simulink model "main_sim_adapt"  (Simulink 7.2)
settings: Solver=ode2  SolverMode=SingleTasking  StartTime=0.0  StopTime=tsim_max  FixedStep=dtsim  RelTol=1e-3
StopFcn:
  | %mkplt
undefined symbols (not defined in the file): aero_surf_qbar_off, aero_surf_qbar_on, assertion_time, att_type, att_type_numbers, bb_ellipsoid, bb_params, compute_all_rate_cols, compute_all_vel_cols, constants, cosA, DiscIntNeverNeededParam, dtsim, E_rwy, eow_boundary, full_surf_llim, full_surf_ulim, gain_set, gain_var_struct, in_exsig_vecin, in_exsig_vecout, MACH, MACH_att_fb, MACH_gain_mat, MACH_mass_IC, MACH_pos_IC, MACH_pqr_Bmat_IC, MACH_pqr_IC, MACH_pqr_u_IC, MACH_quat_IC, MACH_throttle_IC, MACH_U_nom_IC, MACH_vel_Bmat_IC, MACH_vel_cvdnom_IC, MACH_vel_IC, MACH_vel_uold_IC, max_LOS_rate, modes, N_rwy, pos, rcs_cvddes_thresh, reset_camcmd_on_entry, sinA, target_pos_IC, target_range_blind, target_range_detect, target_range_homing, target_vel_IC, trac_params, u_llim, u_ulim, use_auto_att_type, use_eow_as_iv, use_nav, use_pos_fltpath_lim, use_throt_estimate, use_variable_mass, use_wind_est, vel, vel_cmd_ramp_time ... (+1)
libraries: simulink x32, mach_lib x26, utility_lib x24, model_lib x15, simulink_need_slupdate x8, models x6
(part 5 of 5)

== system main_sim_adapt/claw_main/vel_loops/set di params/compute dc_fltpath ==
  NEh_dot_fltpath : Inport  OutDataType=sfix(16)  OutScaling=2^0
  Gain : Gain  Gain=repmat([1 1 -1],3,1)  ParameterDataType=sfix(16)  ParameterScaling=2^0  OutDataType=sfix(16)  OutScaling=2^0
  Gain1 : Gain  Gain=[1 1 -1]  ParameterDataType=sfix(16)  ParameterScaling=2^0  OutDataType=sfix(16)  OutScaling=2^0
  Reshape : Reshape  OutputDimensionality=Customize  OutputDimensions=[3 3]
  Terminator : Terminator
  vec2dc : utility_lib/vec2dc  SystemSampleTime=-1
  dc_fltpath : Outport  OutDataType=sfix(16)  OutScaling=2^0
  wires:
  vec2dc/1 -> Reshape/1
  Reshape/1 -> Gain/1
  Gain1/1 -> vec2dc/1
  vec2dc/2 -> Terminator/1
  Gain/1 -> dc_fltpath/1
  NEh_dot_fltpath/1 -> Gain1/1

== system main_sim_adapt/claw_main/vel_loops/set di params/throttle limits ==
  full_surf : Inport  OutDataType=sfix(16)  OutScaling=2^0
  throt_old : Inport  Port=2  OutDataType=sfix(16)  OutScaling=2^0
  Bus Creator : BusCreator
  Bus Selector1 : BusSelector  OutputSignals=full_surf_ulim,full_surf_llim,full_surf_urlim,full_surf_lrlim
  Selector{1..2,5..6} (4 alike) : Selector  InputPortWidth=MACH.num_u  IndexOptions=Index vector (dialog)  Indices=MACH.throttle_idx  OutputSizes=1
  rate limit limits : mach_lib/rate limit limits  SystemSampleTime=-1  ulim=MACH.vel_throt_ulim  llim=MACH.vel_throt_llim
  throt_limits : Outport  OutDataType=sfix(16)  OutScaling=2^0
  wires:
  Bus Selector1/1 -> Selector5/1  "<full_surf_ulim>"
  Bus Selector1/2 -> Selector6/1  "<full_surf_llim>"
  full_surf/1 -> Bus Selector1/1
  throt_old/1 -> rate limit limits/1
  Selector5/1 -> rate limit limits/2
  Selector6/1 -> rate limit limits/3
  Bus Creator/1 -> throt_limits/1
  rate limit limits/1 -> Bus Creator/1  "throt_ulim"
  rate limit limits/2 -> Bus Creator/2  "throt_llim"
  Bus Selector1/3 -> Selector1/1  "<full_surf_urlim>"
  Bus Selector1/4 -> Selector2/1  "<full_surf_lrlim>"
  Selector1/1 -> rate limit limits/4, Bus Creator/3  "throt_urlim"
  Selector2/1 -> rate limit limits/5, Bus Creator/4  "throt_lrlim"

== system main_sim_adapt/vehicle_model/target/seeker model/seeker model/cart to polar ==
  note: Avoid division by zero when
      | all errors are exactly zero
  scaling info : Inport  OutDataType=sfix(16)  OutScaling=2^0
  cross_d;vert_d : Inport  Port=2  OutDataType=sfix(16)  OutScaling=2^0
  Abs : Abs
  Bus Selector : BusSelector  OutputSignals=Rground,Rslant
  Constant : Constant  Value=0.0001  OutDataType=sfix(16)  OutScaling=2^0
  Gain1 : Gain  Gain=1./max_LOS_rate  ParameterDataType=sfix(16)  ParameterScaling=2^0  OutDataType=sfix(16)  OutScaling=2^0
  Gain2 : Gain  Gain=[1 -1]  ParameterDataType=sfix(16)  ParameterScaling=2^0  OutDataType=sfix(16)  OutScaling=2^0
  MinMax : MinMax  Function=max  Inputs=3  OutDataType=sfix(16)  OutScaling=2^0
  Mux : Mux  Inputs=2
  Product : Product  Inputs=*/  OutDataType=sfix(16)  OutScaling=2^0  RndMeth=Zero
  LOS_rate : Outport  OutDataType=sfix(16)  OutScaling=2^0
  wires:
  Mux/1 -> MinMax/2
  Gain1/1 -> MinMax/1
  Gain2/1 -> Product/2
  MinMax/1 -> Gain2/1
  Abs/1 -> Gain1/1
  Product/1 -> LOS_rate/1
  cross_d;vert_d/1 -> Product/1, Abs/1
  scaling info/1 -> Bus Selector/1
  Bus Selector/1 -> Mux/1  "<Rground>"
  Bus Selector/2 -> Mux/2  "<Rslant>"
  Constant/1 -> MinMax/3

== system main_sim_adapt/claw_main/input processing/mode dependent stick processing/att rate cmd/also reset att on att_type change ==
  reset_in : Inport  OutDataType=sfix(16)  OutScaling=2^0
  Detect Change : simulink/Logic and Bit Operations/Detect Change  SystemSampleTime=-1  vinit=0
  Detect Increase : simulink/Logic and Bit Operations/Detect Increase  SystemSampleTime=-1  vinit=0.0
  Logical Operator2 : Logic  Operator=OR  AllPortsSameDT=off
  Logical Operator3 : Logic  Operator=XOR  AllPortsSameDT=off
  Unit Delay : UnitDelay  Orientation=left  SampleTime=MACH.dt
  reset_out : Outport  OutDataType=sfix(16)  OutScaling=2^0
  wires:
  [att_type] -> Detect Change/1
  Detect Change/1 -> Logical Operator2/2
  Detect Increase/1 -> Logical Operator2/1
  Logical Operator2/1 -> Logical Operator3/1
  Logical Operator3/1 -> Unit Delay/1, reset_out/1
  Unit Delay/1 -> Logical Operator3/2
  reset_in/1 -> Detect Increase/1

== system main_sim_adapt/claw_main/input processing/mode dependent stick processing/feed forward/get att_ff ==
  signal_bus : Inport  OutDataType=sfix(16)  OutScaling=2^0
  Bus Selector : BusSelector  OutputSignals=x_est.uvw,y_meas.accels_cg,y_meas.dircos,x_est.e
  Dot Product : simulink/Math Operations/Dot Product  InputSameDT=on  OutDataType=sfix(16)  OutScaling=2^-10  DoSatur=off
  Gain : Gain  Gain=constants.g  ParameterDataType=sfix(16)  ParameterScaling=2^0  OutDataType=sfix(16)  OutScaling=2^0
  MinMax1 : MinMax  Function=max  Inputs=2  OutDataType=sfix(16)  OutScaling=2^0
  Product1 : Product  Inputs=/*  OutDataType=sfix(16)  OutScaling=2^0  RndMeth=Zero
  Sum2 : Sum  Inputs=|++  OutDataType=sfix(16)  OutScaling=2^0
  V x a : utility_lib/cross product  SystemSampleTime=-1
  down vector : Selector  InputPortWidth=9  IndexOptions=Index vector (dialog)  Indices=7:9  OutputSizes=1
  geted : utility_lib/geted  SystemSampleTime=-1
  protect for   divide by zero : Constant  Value=0.001^2  OutDataType=sfix(16)  OutScaling=2^0
  att_ff : Outport  OutDataType=sfix(16)  OutScaling=2^0
  wires:
  Product1/1 -> geted/1
  V x a/1 -> Product1/2
  signal_bus/1 -> Bus Selector/1
  Bus Selector/1 -> V x a/1, Dot Product/1, Dot Product/2  "<uvw>"
  Bus Selector/4 -> geted/2  "<e>"
  protect for   divide by zero/1 -> MinMax1/2
  MinMax1/1 -> Product1/1
  Sum2/1 -> V x a/2
  geted/1 -> att_ff/1
  Bus Selector/3 -> down vector/1  "<dircos>"
  down vector/1 -> Gain/1
  Gain/1 -> Sum2/2
  Bus Selector/2 -> Sum2/1  "<accels_cg>"
  Dot Product/1 -> MinMax1/1

== system main_sim_adapt/claw_main/input processing/mode dependent stick processing/feed forward/lookup using  energy over weight ==
  eow_idx : Inport  OutDataType=sfix(16)  OutScaling=2^0
  Constant1 : Constant  Value=int32(0:2)  OutDataType=sfix(16)  OutScaling=2^0
  Constant2 : Constant  Value=int32(0:2)  OutDataType=sfix(16)  OutScaling=2^0
  Interpolation (n-D) using PreLookup for acc : simulink_need_slupdate/Interpolation (n-D) using PreLookup  numDimsPopupSelect=2  explicitNumDims=2  table=tbl_acc_eow  interpMethod=Linear  extrapMethod=Linear  rangeErrorMode=None  NumSelectionDims=1
  Interpolation (n-D) using PreLookup for vel : simulink_need_slupdate/Interpolation (n-D) using PreLookup  numDimsPopupSelect=2  explicitNumDims=2  table=tbl_vel_eow  interpMethod=Linear  extrapMethod=Linear  rangeErrorMode=None  NumSelectionDims=1
  pos_ff : Outport  OutDataType=sfix(16)  OutScaling=2^0
  vel_ff : Outport  Port=2  OutDataType=sfix(16)  OutScaling=2^0
  wires:
  Interpolation (n-D) using PreLookup for vel/1 -> pos_ff/1
  Interpolation (n-D) using PreLookup for acc/1 -> vel_ff/1
  eow_idx/1 -> Interpolation (n-D) using PreLookup for vel/1, Interpolation (n-D) using PreLookup for acc/1
  Constant1/1 -> Interpolation (n-D) using PreLookup for vel/2
  Constant2/1 -> Interpolation (n-D) using PreLookup for acc/2

== system main_sim_adapt/claw_main/input processing/mode dependent stick processing/feed forward/lookup using X   ==
  X_idx : Inport  OutDataType=sfix(16)  OutScaling=2^0
  Constant1 : Constant  Value=int32(0:2)  OutDataType=sfix(16)  OutScaling=2^0
  Constant2 : Constant  Value=int32(0:2)  OutDataType=sfix(16)  OutScaling=2^0
  Interpolation (n-D) using PreLookup for acc : simulink_need_slupdate/Interpolation (n-D) using PreLookup  numDimsPopupSelect=2  explicitNumDims=2  table=tbl_acc_X  interpMethod=Linear  extrapMethod=Linear  rangeErrorMode=None  NumSelectionDims=1
  Interpolation (n-D) using PreLookup for vel : simulink_need_slupdate/Interpolation (n-D) using PreLookup  numDimsPopupSelect=2  explicitNumDims=2  table=tbl_vel_X  interpMethod=Linear  extrapMethod=Linear  rangeErrorMode=None  NumSelectionDims=1
  pos_ff : Outport  OutDataType=sfix(16)  OutScaling=2^0
  vel_ff : Outport  Port=2  OutDataType=sfix(16)  OutScaling=2^0
  wires:
  X_idx/1 -> Interpolation (n-D) using PreLookup for vel/1, Interpolation (n-D) using PreLookup for acc/1
  Interpolation (n-D) using PreLookup for vel/1 -> pos_ff/1
  Interpolation (n-D) using PreLookup for acc/1 -> vel_ff/1
  Constant1/1 -> Interpolation (n-D) using PreLookup for vel/2
  Constant2/1 -> Interpolation (n-D) using PreLookup for acc/2

== system main_sim_adapt/claw_main/input processing/mode dependent stick processing/set command selection switches/modify for accel cmd submode ==
  select_cmd_in : Inport  OutDataType=sfix(16)  OutScaling=2^0
  accel_cmd_sw : Inport  Port=2  OutDataType=sfix(16)  OutScaling=2^0
  Assignment : Assignment  IndexOptions=Index vector (dialog)  Indices=[1 2 4]  OutputSizes=[1 1]
  Assignment1 : Assignment  IndexOptions=Index vector (dialog)  Indices=[1 2 4]  OutputSizes=[1 1]
  Bus Assignment : BusAssignment  AssignedSignals=vel,pos
  Bus Selector : BusSelector  OutputSignals=vel
  Bus Selector1 : BusSelector  OutputSignals=pos
  Selector1 : Selector  InputPortWidth=4  IndexOptions=Index vector (dialog)  Indices=[1 2 4]  OutputSizes=1
  Selector2 : Selector  InputPortWidth=4  IndexOptions=Index vector (dialog)  Indices=[1 2 4]  OutputSizes=1
  Switch : Switch  Threshold=0.5
  Switch1 : Switch  Threshold=0.5
  command current pos : Constant  Value=0  OutDataType=sfix(16)  OutScaling=2^0
  command current vel : Constant  Value=0  OutDataType=sfix(16)  OutScaling=2^0
  select_cmd : Outport  OutDataType=sfix(16)  OutScaling=2^0
  wires:
  select_cmd_in/1 -> Bus Assignment/1, Bus Selector/1, Bus Selector1/1
  accel_cmd_sw/1 -> Switch/2, Switch1/2
  Bus Selector/1 -> Selector1/1, Assignment/1  "<vel>"
  command current vel/1 -> Switch/1
  Selector1/1 -> Switch/3
  Switch/1 -> Assignment/2
  Assignment/1 -> Bus Assignment/2
  Bus Assignment/1 -> select_cmd/1
  Bus Selector1/1 -> Selector2/1, Assignment1/1  "<pos>"
  command current pos/1 -> Switch1/1
  Selector2/1 -> Switch1/3
  Switch1/1 -> Assignment1/2
  Assignment1/1 -> Bus Assignment/3

== system main_sim_adapt/claw_main/input processing/mode dependent stick processing/use table lookup pos cmds/use E/W to get pos cmds ==
  eow_idx : Inport  OutDataType=sfix(16)  OutScaling=2^0
  Constant1 : Constant  Value=int32(0:2)  OutDataType=sfix(16)  OutScaling=2^0
  Interpolation (n-D) using PreLookup : simulink_need_slupdate/Interpolation (n-D) using PreLookup  numDimsPopupSelect=2  explicitNumDims=2  table=tbl_pos_eow  interpMethod=Linear  extrapMethod=Linear  rangeErrorMode=None  NumSelectionDims=1
  pos_cmd_eow : Outport  OutDataType=sfix(16)  OutScaling=2^0
  wires:
  Interpolation (n-D) using PreLookup/1 -> pos_cmd_eow/1
  eow_idx/1 -> Interpolation (n-D) using PreLookup/1
  Constant1/1 -> Interpolation (n-D) using PreLookup/2

== system main_sim_adapt/claw_main/input processing/mode dependent stick processing/use table lookup pos cmds/use X to get pos cmds ==
  note: Note: When X is used as the independent variable
      | the trajectory is in a vertical plane and Y=0
  X_idx : Inport  OutDataType=sfix(16)  OutScaling=2^0
  X : Inport  Port=2  OutDataType=sfix(16)  OutScaling=2^0
  Constant1 : Constant  Value=E_rwy  OutDataType=sfix(16)  OutScaling=2^0
  Constant3 : Constant  Value=N_rwy  OutDataType=sfix(16)  OutScaling=2^0
  Constant4 : Constant  Value=cosA  OutDataType=sfix(16)  OutScaling=2^0
  Constant5 : Constant  Value=sinA  OutDataType=sfix(16)  OutScaling=2^0
  Interpolation (n-D) using PreLookup for h : simulink_need_slupdate/Interpolation (n-D) using PreLookup  numDimsPopupSelect=1  explicitNumDims=2  table=tbl_hofX  interpMethod=Linear  extrapMethod=Linear  rangeErrorMode=None  NumSelectionDims=0
  Mux : Mux  Inputs=3
  Product3 : Product  OutDataType=sfix(16)  OutScaling=2^0  RndMeth=Zero
  Product4 : Product  OutDataType=sfix(16)  OutScaling=2^0  RndMeth=Zero
  Sum4 : Sum  Inputs=++|  OutDataType=sfix(16)  OutScaling=2^0
  Sum5 : Sum  Inputs=|++  OutDataType=sfix(16)  OutScaling=2^0
  pos_cmd_X : Outport  OutDataType=sfix(16)  OutScaling=2^0
  wires:
  X_idx/1 -> Interpolation (n-D) using PreLookup for h/1
  Interpolation (n-D) using PreLookup for h/1 -> Mux/3
  Mux/1 -> pos_cmd_X/1
  Constant4/1 -> Product4/1
  Constant5/1 -> Product3/1
  Sum4/1 -> Mux/1
  Product4/1 -> Sum4/2
  Constant3/1 -> Sum4/1
  Sum5/1 -> Mux/2
  Product3/1 -> Sum5/1
  Constant1/1 -> Sum5/2
  X/1 -> Product4/2, Product3/2

== system main_sim_adapt/claw_main/input processing/set control parameters/accel submode setup/NED_dd/vchigam_dot ==
  case : Inport  OutDataType=sfix(16)  OutScaling=2^0
  signal_bus : Inport  Port=2  OutDataType=sfix(16)  OutScaling=2^0
  Action Port : ActionPort  ActionType=case
  Bus Selector3 : BusSelector  OutputSignals=cmd_bus.autopilot_cmd
  Gain : Gain  Gain=[1 1 1]  ParameterDataType=sfix(16)  ParameterScaling=2^0  OutDataType=sfix(16)  OutScaling=2^0
  Selector : Selector  InputPortWidth=4  IndexOptions=Index vector (dialog)  Indices=[1 2 4]  OutputSizes=1
  Signal Conversion : SignalConversion  ConversionOutput=Contiguous copy
  accel_cmd_sw : Outport  OutDataType=sfix(16)  OutScaling=2^0  InitialOutput=zeros(3,1)
  accel_cmd : Outport  Port=2  OutDataType=sfix(16)  OutScaling=2^0  InitialOutput=zeros(3,1)
  wires:
  signal_bus/1 -> Bus Selector3/1
  Bus Selector3/1 -> Selector/1  "<autopilot_cmd>"
  Selector/1 -> Signal Conversion/1
  case/1 -> Gain/1
  Gain/1 -> accel_cmd_sw/1
  Signal Conversion/1 -> accel_cmd/1

== system main_sim_adapt/claw_main/input processing/set control parameters/accel submode setup/homing ==
  signal_bus : Inport  OutDataType=sfix(16)  OutScaling=2^0
  Action Port : ActionPort  ActionType=case
  Bus Selector3 : BusSelector  OutputSignals=y_meas.seeker.aux_info.Rslant,y_meas.seeker.LOS_rate
  Compare To Constant : simulink/Logic and Bit Operations/Compare To Constant  SystemSampleTime=-1  relop=<=  const=target_range_homing  LogicOutDataTypeMode=boolean  ZeroCross=off
  Compare To Constant1 : simulink/Logic and Bit Operations/Compare To Constant  SystemSampleTime=-1  relop=<=  const=target_range_detect  LogicOutDataTypeMode=boolean  ZeroCross=off
  Compare To Constant2 : simulink/Logic and Bit Operations/Compare To Constant  SystemSampleTime=-1  relop=>=  const=target_range_blind  LogicOutDataTypeMode=boolean  ZeroCross=off
  Constant2 : Constant  Value=0  OutDataType=sfix(16)  OutScaling=2^0
  Data Type Conversion : DataTypeConversion  OutDataTypeMode=double  OutDataType=sfix(16)  OutScaling=2^0  OutDataTypeStr=double
  Gain : Gain  Gain=2  ParameterDataType=sfix(16)  ParameterScaling=2^0  OutDataType=sfix(16)  OutScaling=2^0  OutDataTypeStr=Inherit: Inherit via back propagation
  Logical Operator2 : Logic  AllPortsSameDT=off
  Mux : Mux  Inputs=2
  Mux1 : Mux  Inputs=2
  Product3 : Product  OutDataType=sfix(16)  OutScaling=2^0  RndMeth=Zero
  Selector3 : Selector  InputPortWidth=2  IndexOptions=Index vector (dialog)  Indices=[1 1 2]  OutputSizes=1
  azimuth_d/elevation_d gain : Gain  Gain=MACH.K_pn  ParameterDataType=sfix(16)  ParameterScaling=2^0  OutDataType=sfix(16)  OutScaling=2^0
  accel_cmd_sw : Outport  OutDataType=sfix(16)  OutScaling=2^0  InitialOutput=zeros(3,1)
  accel_cmd : Outport  Port=2  OutDataType=sfix(16)  OutScaling=2^0  InitialOutput=zeros(3,1)
  wires:
  Bus Selector3/1 -> Compare To Constant/1, Compare To Constant1/1, Compare To Constant2/1  "<Rslant>"
  Compare To Constant1/1 -> Mux/1
  Compare To Constant/1 -> Mux/2
  Mux/1 -> Logical Operator2/1, Selector3/1
  Compare To Constant2/1 -> Logical Operator2/2
  Selector3/1 -> Data Type Conversion/1
  signal_bus/1 -> Bus Selector3/1
  Bus Selector3/2 -> Product3/2  "<LOS_rate>"
  Product3/1 -> azimuth_d/elevation_d gain/1
  Logical Operator2/1 -> Product3/1  "PN_active"
  Constant2/1 -> Mux1/1
  azimuth_d/elevation_d gain/1 -> Mux1/2
  Gain/1 -> accel_cmd_sw/1
  Mux1/1 -> accel_cmd/1
  Data Type Conversion/1 -> Gain/1

== system main_sim_adapt/claw_main/input processing/set control parameters/accel submode setup/normal vel desdyn ==
  Action Port : ActionPort  ActionType=default
  Constant1 : Constant  Value=zeros(3,1)  OutDataType=sfix(16)  OutScaling=2^0
  Constant2 : Constant  Value=zeros(3,1)  OutDataType=sfix(16)  OutScaling=2^0
  accel_cmd_sw : Outport  OutDataType=sfix(16)  OutScaling=2^0  InitialOutput=zeros(3,1)
  accel_cmd : Outport  Port=2  OutDataType=sfix(16)  OutScaling=2^0  InitialOutput=zeros(3,1)
  wires:
  Constant1/1 -> accel_cmd/1
  Constant2/1 -> accel_cmd_sw/1

== system main_sim_adapt/claw_main/input processing/set control parameters/select gains/mux to bus ==
  mux_in : Inport  OutDataType=sfix(16)  OutScaling=2^0
  Bus Creator : BusCreator  Inputs=16
  Demux : Demux  Outputs=[4;4;4;4;3;3;3;3;3;3;3;3;3;3;3;3]
  bus_out : Outport  OutDataType=sfix(16)  OutScaling=2^0
  wires:
  mux_in/1 -> Demux/1
  Bus Creator/1 -> bus_out/1
  Demux/1 -> Bus Creator/1  "MACH_att_Kaw"
  Demux/2 -> Bus Creator/2  "MACH_att_Kb"
  Demux/3 -> Bus Creator/3  "MACH_att_Kf"
  Demux/4 -> Bus Creator/4  "MACH_att_Ki"
  Demux/5 -> Bus Creator/5  "MACH_pos_Kaw"
  Demux/6 -> Bus Creator/6  "MACH_pos_Kb"
  Demux/7 -> Bus Creator/7  "MACH_pos_Kf"
  Demux/8 -> Bus Creator/8  "MACH_pos_Ki"
  Demux/9 -> Bus Creator/9  "MACH_pqr_Kaw"
  Demux/10 -> Bus Creator/10  "MACH_pqr_Kb"
  Demux/11 -> Bus Creator/11  "MACH_pqr_Kf"
  Demux/12 -> Bus Creator/12  "MACH_pqr_Ki"
  Demux/13 -> Bus Creator/13  "MACH_vel_Kaw"
  Demux/14 -> Bus Creator/14  "MACH_vel_Kb"
  Demux/15 -> Bus Creator/15  "MACH_vel_Kf"
  Demux/16 -> Bus Creator/16  "MACH_vel_Ki"

== system main_sim_adapt/claw_main/input processing/set control parameters/set rate di params/fix aero surfs when low qbar ==
  pqr_u_ulim_in : Inport  OutDataType=sfix(16)  OutScaling=2^0
  pqr_u_llim_in : Inport  Port=2  OutDataType=sfix(16)  OutScaling=2^0
  low_qbar : Inport  Port=3  OutDataType=sfix(16)  OutScaling=2^0
  pqr_u_pref : Inport  Port=4  OutDataType=sfix(16)  OutScaling=2^0
  Assignment : Assignment  IndexOptions=Index vector (dialog)  Indices=MACH.vane_idx  OutputSizes=[1 1]
  Assignment1 : Assignment  IndexOptions=Index vector (dialog)  Indices=MACH.vane_idx  OutputSizes=[1 1]
  MinMax : MinMax  Inputs=2  OutDataType=sfix(16)  OutScaling=2^0
  MinMax1 : MinMax  Function=max  Inputs=2  OutDataType=sfix(16)  OutScaling=2^0
  Multiport Switch1 : MultiPortSwitch  Inputs=2  zeroidx=on  SaturateOnIntegerOverflow=on
  Multiport Switch2 : MultiPortSwitch  Inputs=2  zeroidx=on  SaturateOnIntegerOverflow=on
  Selector1 : Selector  InputPortWidth=MACH.pqr_num_u  IndexOptions=Index vector (dialog)  Indices=MACH.vane_idx  OutputSizes=1
  Selector2 : Selector  InputPortWidth=MACH.pqr_num_u  IndexOptions=Index vector (dialog)  Indices=MACH.vane_idx  OutputSizes=1
  Selector6 : Selector  InputPortWidth=MACH.pqr_num_u  IndexOptions=Index vector (dialog)  Indices=MACH.vane_idx  OutputSizes=1
  pqr_u_ulim : Outport  OutDataType=sfix(16)  OutScaling=2^0
  pqr_u_llim : Outport  Port=2  OutDataType=sfix(16)  OutScaling=2^0
  wires:
  low_qbar/1 -> Multiport Switch1/1, Multiport Switch2/1
  pqr_u_pref/1 -> Selector6/1
  pqr_u_ulim_in/1 -> Assignment/1, Multiport Switch1/2, Selector1/1
  pqr_u_llim_in/1 -> Assignment1/1, Multiport Switch2/2, Selector2/1
  Multiport Switch1/1 -> pqr_u_ulim/1
  Assignment/1 -> Multiport Switch1/3
  Multiport Switch2/1 -> pqr_u_llim/1
  Assignment1/1 -> Multiport Switch2/3
  Selector1/1 -> MinMax/1
  Selector6/1 -> MinMax/2
  MinMax/1 -> MinMax1/1
  Selector2/1 -> MinMax1/2
  MinMax1/1 -> Assignment/2, Assignment1/2

== system main_sim_adapt/claw_main/input processing/set control parameters/set rate di params/select u_pref ==
  note: "from outer" not yet implemented
  note: "test" not yet implemented
  note: Use schedule if configured and qbar is low
  low_qbar : Inport  OutDataType=sfix(16)  OutScaling=2^0
  aero_env_est : Inport  Port=2  OutDataType=sfix(16)  OutScaling=2^0
  full_surf : Inport  Port=3  OutDataType=sfix(16)  OutScaling=2^0
  Bus Selector4 : BusSelector  OutputSignals=full_surf_pref_select,full_surf_pref,full_surf_pref_wght,full_surf_cmd
  Constant2 : Constant  Value=MACH.pqr_wght_u_pref_high  OutDataType=sfix(16)  OutScaling=2^0
  Demux : Demux  Outputs=2
  From Workspace : FromWorkspace  VariableName=use_preference_schedule_fw  SampleTime=MACH.dt  Interpolate=off  OutputAfterFinalValue=Holding final value
  Logical Operator : Logic  AllPortsSameDT=off
  Logical Operator1 : Logic  Operator=NOT  AllPortsSameDT=off
  MinMax : MinMax  Function=max  Inputs=2  OutDataType=sfix(16)  OutScaling=2^0
  Multiport Switch : MultiPortSwitch  Inputs=5  zeroidx=on
  Mux{,1..3} (4 alike) : Mux  Inputs=2
  Selector{1..3,5} (4 alike) : Selector  InputPortWidth=MACH.num_u  IndexOptions=Index vector (dialog)  Indices=MACH.pqr_u_idx  OutputSizes=1
  preference schedule : model_lib/no preference schedule  SystemSampleTime=-1
  u_pref : Outport  OutDataType=sfix(16)  OutScaling=2^0
  wght_u_pref : Outport  Port=2  OutDataType=sfix(16)  OutScaling=2^0
  wires:
  Selector1/1 -> preference schedule/1, Mux/1
  Selector2/1 -> preference schedule/2, Mux/2
  Mux/1 -> Multiport Switch/2, Multiport Switch/5, Multiport Switch/6
  Multiport Switch/1 -> Demux/1
  Demux/1 -> u_pref/1
  Demux/2 -> wght_u_pref/1
  aero_env_est/1 -> preference schedule/3
  preference schedule/1 -> Mux1/1
  preference schedule/2 -> Mux1/2
  Mux1/1 -> Multiport Switch/3
  low_qbar/1 -> Logical Operator1/1
  full_surf/1 -> Bus Selector4/1
  Mux2/1 -> Multiport Switch/4
  Constant2/1 -> Mux2/2
  Selector5/1 -> Mux2/1
  Bus Selector4/1 -> Selector3/1  "<full_surf_pref_select>"
  Bus Selector4/2 -> Selector1/1  "<full_surf_pref>"
  Bus Selector4/3 -> Selector2/1  "<full_surf_pref_wght>"
  Bus Selector4/4 -> Selector5/1  "<full_surf_cmd>"
  Selector3/1 -> MinMax/2
  Mux3/1 -> Multiport Switch/1
  MinMax/1 -> Mux3/1, Mux3/2
  Logical Operator1/1 -> Logical Operator/2
  From Workspace/1 -> Logical Operator/1
  Logical Operator/1 -> MinMax/1

== system main_sim_adapt/claw_main/state est/wind estimator/wind estimate/rate and  position limits ==
  w_est : Inport  OutDataType=sfix(16)  OutScaling=2^0
  Constant : Constant  Value=MACH.est_w_ulim  OutDataType=sfix(16)  OutScaling=2^0
  Constant1 : Constant  Value=MACH.est_w_llim  OutDataType=sfix(16)  OutScaling=2^0
  Constant2 : Constant  Value=MACH.est_w_urlim  OutDataType=sfix(16)  OutScaling=2^0
  Constant3 : Constant  Value=MACH.est_w_lrlim  OutDataType=sfix(16)  OutScaling=2^0
  MinMax : MinMax  Function=max  Inputs=2  OutDataType=sfix(16)  OutScaling=2^0  SaturateOnIntegerOverflow=on  InputSameDT=on
  MinMax1 : MinMax  Inputs=2  OutDataType=sfix(16)  OutScaling=2^0  SaturateOnIntegerOverflow=on  InputSameDT=on
  Unit Delay : UnitDelay  SampleTime=-1
  limit computation : mach_lib/limit computation  SystemSampleTime=-1
  w_est_lim : Outport  OutDataType=sfix(16)  OutScaling=2^0
  wires:
  w_est/1 -> MinMax1/1
  Unit Delay/1 -> limit computation/1
  MinMax1/1 -> MinMax/1
  limit computation/1 -> MinMax1/2
  Constant/1 -> limit computation/3
  Constant1/1 -> limit computation/2
  Constant2/1 -> limit computation/4
  MinMax/1 -> w_est_lim/1, Unit Delay/1
  limit computation/2 -> MinMax/2
  Constant3/1 -> limit computation/5

== system main_sim_adapt/claw_main/vel_loops/B matrix comp/B matrix comp/compute cvd_pert ==
  note: Note: this computation of NEh accelerations
      | assumes that pqr = 0
  x : Inport  OutDataType=sfix(16)  OutScaling=2^0
  u : Inport  Port=2  OutDataType=sfix(16)  OutScaling=2^0
  w_est : Inport  Port=3  OutDataType=sfix(16)  OutScaling=2^0
  Bus Selector : BusSelector  OutputSignals=dircos
  Gain : Gain  Gain=[1 1 -1]  ParameterDataType=sfix(16)  ParameterScaling=2^0  OutDataType=sfix(16)  OutScaling=2^0  SaturateOnIntegerOverflow=on  OutDataTypeStr=Inherit: Same as input  ParamDataTypeStr=Inherit: Same as input
  Math Function : Math  Operator=transpose  OutDataType=sfix(16)  OutScaling=2^0  SaturateOnIntegerOverflow=on
  Product : Product  Multiplication=Matrix(*)  OutDataType=sfix(16)  OutScaling=2^0  SaturateOnIntegerOverflow=on  InputSameDT=on  OutDataTypeStr=Inherit: Same as first input
  Reshape : Reshape  OutputDimensionality=Customize  OutputDimensions=[3,3]
  cl model : models/gtm-obac  SystemSampleTime=-1
  uvw_dot : Selector  InputPortWidth=MACH.num_x  IndexOptions=Index vector (dialog)  Indices=MACH.uvw_idx  OutputSizes=1
  cvd : Outport  OutDataType=sfix(16)  OutScaling=2^0
  wires:
  uvw_dot/1 -> Product/2
  x/1 -> cl model/1
  Reshape/1 -> Math Function/1
  Math Function/1 -> Product/1
  Product/1 -> Gain/1
  Gain/1 -> cvd/1
  Bus Selector/1 -> Reshape/1  "<dircos>"
  u/1 -> cl model/2
  w_est/1 -> cl model/3
  cl model/1 -> uvw_dot/1
  cl model/2 -> Bus Selector/1

== system main_sim_adapt/claw_main/vel_loops/B matrix comp/B matrix comp/compute perturbed XU ==
  X_in : Inport  OutDataType=sfix(16)  OutScaling=2^0
  U_in : Inport  Port=2  OutDataType=sfix(16)  OutScaling=2^0
  D_in : Inport  Port=3  OutDataType=sfix(16)  OutScaling=2^0
  camcmd : Inport  Port=4  OutDataType=sfix(16)  OutScaling=2^0
  NEh_dot : Inport  Port=5  OutDataType=sfix(16)  OutScaling=2^0
  Assignment1 : Assignment  IndexOptions=Index vector (dialog)  Indices=MACH.throttle_idx  OutputSizes=[1 1]
  Assignment2 : Assignment  IndexOptions=Index vector (dialog)  Indices=[ MACH.quat_idx MACH.uvw_idx]  OutputSizes=[1 1]
  Demux1 : Demux  Outputs=[ 2 MACH.num_u_throt ]
  Gain : Gain  Gain=[1 1 -1]  ParameterDataType=sfix(16)  ParameterScaling=2^0  OutDataType=sfix(16)  OutScaling=2^0  SaturateOnIntegerOverflow=on  OutDataTypeStr=Inherit: Same as input  ParamDataTypeStr=Inherit: Same as input
  Mux : Mux  Inputs=[ 2 1 ]
  Mux1 : Mux  Inputs=2
  Product1 : Product  Multiplication=Matrix(*)  OutDataType=sfix(16)  OutScaling=2^0  SaturateOnIntegerOverflow=on  OutDataTypeStr=Inherit: Same as first input
  Reshape1 : Reshape  OutputDimensionality=Customize  OutputDimensions=[3,3]
  Selector1 : Selector  InputPortWidth=MACH.num_x  IndexOptions=Index vector (dialog)  Indices=MACH.quat_idx  OutputSizes=1
  att2dc : utility_lib/att2dc  SystemSampleTime=-1
  dc2e_ref : utility_lib/dc2e_ref  SystemSampleTime=-1
  X_out : Outport  OutDataType=sfix(16)  OutScaling=2^0
  U_out : Outport  Port=2  OutDataType=sfix(16)  OutScaling=2^0
  wires:
  Mux/1 -> att2dc/1
  Demux1/2 -> Assignment1/2  "throttle"
  D_in/1 -> Demux1/1
  U_in/1 -> Assignment1/1
  X_in/1 -> Assignment2/1, Selector1/1
  Assignment1/1 -> U_out/1
  camcmd/1 -> Mux/2
  Demux1/1 -> Mux/1
  NEh_dot/1 -> Gain/1
  Reshape1/1 -> Product1/1
  Assignment2/1 -> X_out/1
  att2dc/1 -> Reshape1/1, dc2e_ref/1
  dc2e_ref/1 -> Mux1/1  "e"
  Gain/1 -> Product1/2  "NED_dot"
  Selector1/1 -> dc2e_ref/2
  Product1/1 -> Mux1/2  "uvw"
  Mux1/1 -> Assignment2/2

== system main_sim_adapt/claw_main/vel_loops/B matrix comp/B matrix comp/pert_comp ==
  col : Inport  OutDataType=sfix(16)  OutScaling=2^0
  d_nom : Inport  Port=2  OutDataType=sfix(16)  OutScaling=2^0
  params : Inport  Port=3  OutDataType=sfix(16)  OutScaling=2^0
  Bus Selector : BusSelector  OutputSignals=u_ulim,u_llim
  Constant2 : Constant  Value=diag(MACH.vel_u_pert)  OutDataType=sfix(16)  OutScaling=2^0
  pick +/- pert : mach_lib/pick +//- pert  SystemSampleTime=-1  num_u=MACH.vel_num_u
  d_pert : Outport  OutDataType=sfix(16)  OutScaling=2^0
  d_div : Outport  Port=2  OutDataType=sfix(16)  OutScaling=2^0
  wires:
  pick +/- pert/2 -> d_div/1  "scalar pert value"
  d_nom/1 -> pick +/- pert/2
  pick +/- pert/1 -> d_pert/1
  col/1 -> pick +/- pert/1
  Constant2/1 -> pick +/- pert/5
  params/1 -> Bus Selector/1
  Bus Selector/1 -> pick +/- pert/3  "<u_ulim>"
  Bus Selector/2 -> pick +/- pert/4  "<u_llim>"

== system main_sim_adapt/claw_main/vel_loops/convert accel_cmd to NED_dd_cmd/vchigam_dot cmd/polar to cart ==
  note: Note: these are actually Vground and Vslant
  scaling_info : Inport  OutDataType=sfix(16)  OutScaling=2^0
  vchigam_dot_cmd : Inport  Port=2  OutDataType=sfix(16)  OutScaling=2^0
  Bus Selector : BusSelector  OutputSignals=Rground,Rslant
  Demux : Demux  Outputs=[1 2]
  Gain1 : Gain  Gain=[1 -1]  ParameterDataType=sfix(16)  ParameterScaling=2^0  OutDataType=sfix(16)  OutScaling=2^0
  Mux : Mux  Inputs=2
  Mux1 : Mux  Inputs=2
  Product3 : Product  OutDataType=sfix(16)  OutScaling=2^0  RndMeth=Zero
  along_dd;cross_dd;vert_dd : Outport  OutDataType=sfix(16)  OutScaling=2^0
  wires:
  scaling_info/1 -> Bus Selector/1
  Mux/1 -> Gain1/1
  vchigam_dot_cmd/1 -> Demux/1
  Bus Selector/1 -> Mux/1  "<Rground>"
  Bus Selector/2 -> Mux/2  "<Rslant>"
  Gain1/1 -> Product3/2
  Demux/2 -> Product3/1
  Demux/1 -> Mux1/1
  Product3/1 -> Mux1/2
  Mux1/1 -> along_dd;cross_dd;vert_dd/1

== matlab function claw_main/rate_loops/allocation/RCS allocation/Embedded MATLAB Function ==
  data: Bmat input double; wght_cv input double; ulim input double; llim input double; cvd_des input double; rcs_cmd output double; minerr output double; scale output double; cvd_actual output double; err_thresh input double; rcs_use_in input double
function [rcs_cmd, minerr, scale, cvd_actual] = rcs_alloc(Bmat, wght_cv, ulim, llim, cvd_des, err_thresh, rcs_use_in)

rcs_quant = 0;
scale = 1;

nrcs = size(Bmat,2);


if(nrcs == 6)
    % assume fake RCS
    gang_pos = [0 0 0; 0 0 0; 1 1 0; 1 0 0; 0 0 1; 0 1 0];
    gang_neg = [1 1 0; 0 0 1; 0 0 0; 0 1 0; 0 0 0; 1 0 0];

    gain_factor = 1./diag(Bmat*gang_pos);
    rcs_cmd = gang_neg*(gain_factor.*max(0,-cvd_des)) + gang_pos*(gain_factor.*max(0,cvd_des));
    if(rcs_quant > 0)
        rcs_cmd = round(rcs_cmd/rcs_quant)*rcs_quant;
    end
    rcs_cmd = max(min(rcs_cmd,ulim),llim);
    cvd_actual = Bmat*rcs_cmd;
    minerr = norm_vec(cvd_actual - cvd_des);
    
    return
end

rcs_cmd = llim;
cvd_actual = Bmat*rcs_cmd; 
minerr = norm_vec((cvd_actual - cvd_des).*wght_cv);

if(minerr <= err_thresh)
    return
end

Bmat = diag(wght_cv)*Bmat;
cvd_des = wght_cv.*cvd_des;

scale_trial = 1;
normsq_cvd_trial = 0;

powersof2 = 2.^[0:nrcs-1];
bllim = uint32(powersof2*llim);
bulim = uint32(powersof2*ulim);
rcs_use_all = uint32([1:2^nrcs-1]');
rcs_use_tmp = bitor(rcs_use_all,uint32(bllim));
rcs_use_tmp = bitand(rcs_use_tmp,uint32(bulim));
rcs_use = rcs_use_in.*eq(rcs_use_tmp,rcs_use_all);

if(~any(rcs_use))
    return
end

for i = 1:length(rcs_use)
    
    if(~rcs_use(i))
        continue
    end
    
    rcson = double(bitget(uint32(i),1:nrcs))';
    cvd_trial = Bmat*rcson;
    
    % optional scaling
    if(0)
        scale_trial = dot(cvd_des,cvd_trial);
        if(scale_trial < 0)
            continue
        end
        
        normsq_cvd_trial = dot(cvd_trial,cvd_trial);
        if(normsq_cvd_trial <= scale_trial)
            scale_trial = 1;
        else
            scale_trial = dot(cvd_des,cvd_trial)/normsq_cvd_trial;
            cvd_trial = cvd_trial*scale_trial;
        end
    end
    
    cvd_ex = cvd_trial - cvd_des;
    err = norm_vec(cvd_ex);
    if(err < minerr)
        scale = scale_trial;
        rcs_cmd = rcson*scale;
        minerr = err;
        cvd_actual = cvd_trial./wght_cv;
    end
end

function out = norm_vec(in)

out = sqrt(sum(in.^2));

return

== matlab function claw_main/rate_loops/bangbang/Bang Bang ==
  data: bb_params input double; bb_ellipsoid input double; debug_output output double; cvddes output double; dir output double; use_bb output double; att_cvc input double; att_cv input double; timer output double; pqr input double; inertia input double; enable_bb input double; cvddes_lin input double; dir_old input double; use_bb_old input double; timer_old input double
function [debug_output,cvddes,dir,use_bb,timer] = bangbang(bb_params,bb_ellipsoid,att_cvc,att_cv,pqr,inertia,enable_bb,cvddes_lin,dir_old,use_bb_old,timer_old)
% This block supports an embeddable subset of the MATLAB language.
% See the help menu for details. 

dt = bb_params(1) ;
timer_max = bb_params(2) ;
att_thresh = bb_params(3) ;
rate_thresh = bb_params(4) ;
att_diff_thresh = bb_params(5) ;
pp_params = bb_params(6:end) ;

debug_output = zeros(12,1) ;
cvddes = cvddes_lin ;
use_bb = 0 ;
dir = zeros(3,1) ;
timer = timer_old ;

if( ~enable_bb )
    return
end
    
trans = qmpy([1 -1 -1 -1]'.*att_cv,att_cvc) ;

% default is to use dir_old if we were in bangbang last cycle,
% and the timer has not expired
use_dir_old = use_bb_old ;
if( use_dir_old )
    timer = timer + dt ;
    if( timer > timer_max )
        % if timer expires, don't use dir_old
        use_dir_old = 0 ;
    end
end

% compute att using current transformation quat
trans_mag = trans(1) ;
trans_dir = trans(2:4) ;
att = -2*atan2(norm_vec3(trans_dir),trans_mag) ;
att_old = -2*atan2(dir_old'*trans_dir,trans_mag) ;

% choose arbitrary att (and dir) sign to be the same as that computed using
% dir_old.  This is equivalent to making dir_old'*trans_dir positive.
if( att*att_old < 0 )
    att = -att ;
    trans_dir = -trans_dir ;
end

% if we intended to use dir_old, but the angle computed using
% dir_old is significantly different than that derived using the current
% transformation, we will use current dir.
% NOTE: the angle test below works only because att has been adjusted
% to have the same sign as att_old, and both result from atan2 
if( use_dir_old )
    if( abs(att - att_old) > att_diff_thresh )
        use_dir_old = 0 ;
    else
        dir = dir_old ;
        att = att_old ;
    end
end

% check condition to enter (or stay in) bangbang
if( abs(att) > att_thresh )
    use_bb = 1 ;
    
    if( ~use_dir_old )
        dir = trans_dir/norm_vec3(trans_dir) ;
        timer = 0 ;
    end

elseif( max(abs(pqr)) > rate_thresh )
    use_bb = 1 ;
    
    % if small attitude error, set dir based on rates
    if( ~use_dir_old )
        dir = pqr/norm_vec3(pqr) ;
        att = -2*atan2(dir'*trans_dir,trans_mag) ;
        timer = 0 ;
    end
else
    % even though not used, pass dir_old through for in case of ~use_bb
    dir = dir_old ;
    att = att_old ;
end

% Note: cvddes has been set to a default value of cvddes_lin

if( use_bb )
    rate = pqr'*dir ;
    accel_max = get_ellipsoid_scaling(inertia*dir,bb_ellipsoid) ;
    accel_min = -accel_max ;
    pp_params(1) = accel_max ;
    pp_params(2) = accel_min ;
    [outside,accel] = pp(pp_params,att,rate) ;
    
    if( outside <= 1 )
        % use default cvddes (cvddes_lin)
        use_bb = 0 ; 
    else
        % eliminate component of linear command in direction dir
        cvddes = cvddes - (dir'*cvddes)*dir ;
    end
else
    % use default cvddes (cvddes_lin)
    rate = 0 ;
    outside = 0 ;
    accel = 0 ;
end

% saturate command at ellipsoid
blend_lin_claw = cvddes*min(get_ellipsoid_scaling(inertia*cvddes,bb_ellipsoid),1) ;

% add component from bangbang
blend_bb_claw = accel*dir ;
cvddes = blend_lin_claw + blend_bb_claw ;

pp_utQu = 1/get_ellipsoid_scaling(inertia*cvddes,bb_ellipsoid) ;
debug_output = [att;att_old;rate;outside;accel;pp_utQu;blend_bb_claw;blend_lin_claw] ;

if( ~use_bb )
    
    % if not using bangbang reset the timer, and set dir to zero
    timer = 0 ;
    % dir used for cvd_des blending is now zeroed outside of this block,
    % so that dir can be retained through a temporary ~use_bb condition
%     dir = 0*dir ;
end

function r = qmpy(p,q)

p0 = p(1) ;
p1 = p(2) ;
p2 = p(3) ;
p3 = p(4) ;

q0 = q(1) ;
q1 = q(2) ;
q2 = q(3) ;
q3 = q(4) ;

r0 = p0 * q0 - p1 * q1 - p2 * q2 - p3 * q3 ;
r1 = p0 * q1 + p1 * q0 + p2 * q3 - p3 * q2 ;
r2 = p0 * q2 - p1 * q3 + p2 * q0 + p3 * q1 ;
r3 = p0 * q3 + p1 * q2 - p2 * q1 + p3 * q0 ;

r = [ r0 r1 r2 r3 ]' ;

function scale = get_ellipsoid_scaling(dir,ellipsoid)
    scale = 1/max(sqrt(dir'*(ellipsoid*dir)),1e-12) ;

function [outside,accel] = pp(params,att,rate)

% the linear control law is
% accel = ww^2 * ( att_cmd - att ) - 2 * zeta * ww * rate

amax = params(1) ; 
amin = params(2) ; 
ww = params(3) ;  
zeta = params(4) ; 
rate_des1 = params(5) ; 
rate_des2 = params(6) ;

% make switch curves conservative
swcurve_shrink = 1.0 ;

swcurve_pos = 0.5 * rate^2 - swcurve_shrink * amin * att ;
swcurve_neg = 0.5 * rate^2 - swcurve_shrink * amax * att ;

% replace ellipse with parallelogram
% outside = ( ww^2 * att^2 + 2 * zeta * ww * att * rate + rate^2 ) / ( ( 1 - zeta^2 ) * amax^2 / ww^2 ) ;
sx1 = 1 + zeta + 4 * zeta^2 ;
sv1 = -0.5 - 2 * zeta ;
sx2 = 1 - 4 * zeta^2
sv2 = 2 * zeta ;
p1 = [sx1; sv1] ;
p2 = [sx2; sv2] ;

outside = 2*ww/amax*max(abs(([p2+p1 p2-p1]\[att*ww; rate])))
accel = 0 ;

if( outside <= 1 )
    return
end

if( rate > 0 )
    if( swcurve_pos < 0 )
        if( rate < rate_des1 )
            accel = amax ;
        elseif( rate < rate_des2 )
            accel = 0 ;
        else
            accel = amin ;
        end
    else
        accel = amin ;
    end
else
    if( swcurve_neg < 0 )
        if( rate > -rate_des1 )
            accel = amin ;
        elseif( rate > - rate_des2 )
            accel = 0 ;
        else
            accel = amax ;
        end
    else
        accel = amax ;
    end
end


function out = norm_vec3(in)

out = sqrt(in(1)^2 + in(2)^2 + in(3)^2);

return
